simulink model "psbthermal"  (Simulink 6.0)
settings: Solver=ode23tb  StartTime=0.0  StopTime=0.5  MaxStep=50e-6  RelTol=1e-3
InitFcn:
  | powericon('psbinitsys',bdroot);
undefined symbols (not defined in the file or in its folder): D1, Delta
libraries: powerlib2 x31, powerlib_extras x1
settings Model: Creator=rchampag  LastModifiedBy=batserve  ExtModeTrigMode=oneshot  ExtModeArmWhenConnect=off  ExtModeAutoUpdateStatusClock=off
settings DataIOCC: LimitDataPoints=off  SaveOutput=off  SaveTime=off  TimeSaveName=t  SignalLoggingName=sigsOut
settings OptimizationCC: BlockReduction=off  BooleanDataType=off
settings DebuggingCC: CheckExecutionContextPreStartOutputMsg=on  CheckExecutionContextRuntimeOutputMsg=on  SolverPrmCheckMsg=none
settings HardwareCC: TargetUnknown=on

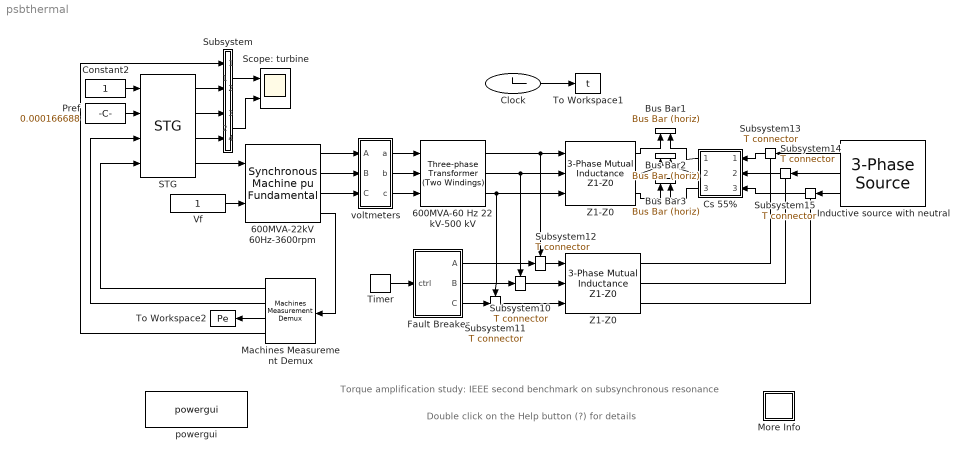
== system psbthermal ==
  note: Torque amplification study:
      | IEEE second benchmark on subsynchronous resonance
  note: Double click on the Help button (?) for details
  600MVA-22kV 60Hz-3600rpm : powerlib2/Machines/Synchronous Machine pu Fundamental  Tag=PoWeRsYsTeMbLoCk  rotorType=Round  x1="[ 600e6  22e3   60 ]"  x2="[  0.0045  0.14  1.51  1.45 ]"  x3="[  0.00096  0.1186 ]"  x4b="[ 0.016  0.132  0.00898  0.411  0.0116  0.0738 ]"  x4="[ 1.1685E-02  0.18167  1.9718E-02  038371 ]"  x5="[ 0.87882   0.176*8   1 ]"  x6="[0  0   0 0 0   0 0 0   0]"  x7=off  x8=[0.6404,0.7127,0.8441,0.9214,0.9956,1.082,1.19,1.316,1.457;0.7,0.7698,0.8872,0.9466,0.9969,1.046,1.1,1.151,1.201]  PSBOutputType=1110  iounits=0  LoadFlowParameters=[1 100000 0 0]
  600MVA-60 Hz 22 kV-500 kV : powerlib2/Elements/Three-phase Transformer (Two Windings)  Tag=PoWeRsYsTeMbLoCk  nominal="[ 600e6   60 ]"  type1=Delta (D1)  params1="[ 22e3  1e-6   0  ]"  type2=Yg  params2="[ 500e3  0.0012   0.12 ]"  ynsat=off  rmag=500  lm=500  sat="[ 0,0  ;  0.005,1.2  ;  1.0,1.4 ]"  hyst=off  matfile='hysteresis'  sif=off  phi0=[ 0.8 , -0.8 , 0.7 ]  initialslopes=[+1 +1 +1]  mesure=None  PSBOutputType=1111
  Bus Bar1 : powerlib2/Connectors/Bus Bar (horiz)  Tag=PoWeRsYsTeMbLoCk  Orientation=up  entrees=2  sorties=0  PSBOutputType=1111111111111111111111111111111111111111111111111111111111111111111111111
  Bus Bar2 : powerlib2/Connectors/Bus Bar (horiz)  Tag=PoWeRsYsTeMbLoCk  Orientation=up  entrees=2  sorties=0  PSBOutputType=1111111111111111111111111111111111111111111111111111111111111111111111111
  Bus Bar3 : powerlib2/Connectors/Bus Bar (horiz)  Tag=PoWeRsYsTeMbLoCk  Orientation=up  entrees=2  sorties=0  PSBOutputType=1111111111111111111111111111111111111111111111111111111111111111111111111
  Clock : Clock
      settings: Decimation=100
  Constant2 : Constant
  Cs 55% : Subsystem  Orientation=left
      mask Display: plot(0,0,100,100,[40,10],[50,50],[90,60],[50,50],[40,40],[20,80],[60,60],[20,80])
  Fault Breaker : Subsystem
  Inductive source with neutral : powerlib2/Electrical Sources/3-Phase Source  Tag=PoWeRsYsTeMbLoCk  Orientation=left  V=500e3  Phi=0  F=60  InternalConnection=Yg  RLoff=off  R=3.5  L=0.1989  Psc=0  Vbase=0  XRratio=0  PSBOutputType=111
  Machines Measurement Demux : powerlib2/Machines/Machines Measurement Demux  Orientation=left  machType=Synchronous  ssm1=on  ssm2=on  ssm3=on  ssm4=on  ssm5=on  ssm6=on  sm1=off  sm2=off  sm3=off  sm4=off  sm5=off  sm6=off  sm7=on  sm8=on  sm9=on  sm10=on  sm11=off  sm115=off  sm12=off  sm13=off  sm14=off  asm1=on  asm2=on  asm3=on  asm4=on  asm5=on  asm6=on  asm7=on  asm8=on  asm9=on  asm10=on  asm11=on  pmsm1=on  pmsm2=on  pmsm3=on  pmsm4=on  pmsm5=on  pmsm6=on  lastType=2
  More Info : Subsystem
      mask Display: disp('?')
  Pref : Constant  Value=0.000166688
  STG : powerlib2/Machines/STG  gentype=Tandem-compound (multi-mass)  reg1="[ 1  0.05    0 ]"  reg2="[ 0.001  0.15 ]"  reg3="[ -0.1  0.1  0.00016668  0.00016668*1.01 ]"  turb1="[ 0  10   3.3   0.5   ]"  turb2="[ 0.5   0.5   0  0 ]"  HA="[  1.5498   0.24894  0  0 ]"  KA="[  83.47  42.702  0  0 ]"  DA="[  0.3104  0.05  0  0 ]*8"  ini1=250.35/555  ini2=[0.000166688,-120.04]
  Scope: turbine : Scope  NumInputPorts=2
      settings: TimeRange=0.5  YMin=-0.9~-70  YMax=0.6~130
  Subsystem : Subsystem
  Subsystem10 : powerlib2/Connectors/T connector  Tag=PoWeRsYsTeMbLoCk  PSBOutputType=1
  Subsystem11 : powerlib2/Connectors/T connector  Tag=PoWeRsYsTeMbLoCk  PSBOutputType=1
  Subsystem12 : powerlib2/Connectors/T connector  Tag=PoWeRsYsTeMbLoCk  PSBOutputType=1
  Subsystem13 : powerlib2/Connectors/T connector  Tag=PoWeRsYsTeMbLoCk  Orientation=left  PSBOutputType=1
  Subsystem14 : powerlib2/Connectors/T connector  Tag=PoWeRsYsTeMbLoCk  Orientation=left  PSBOutputType=1
  Subsystem15 : powerlib2/Connectors/T connector  Tag=PoWeRsYsTeMbLoCk  Orientation=left  PSBOutputType=1
  Timer : powerlib_extras/Control  Blocks/Timer  t="[ 0.022289  0.022289+0.017 ]"  e=[ 1 0 ]
  To Workspace1 : ToWorkspace  VariableName=t  SaveFormat=Array
  To Workspace2 : ToWorkspace  VariableName=Pe  SaveFormat=Array
  Vf : Constant
  Z1-Z0 : powerlib2/Elements/3-Phase Mutual Inductance Z1-Z0  RL1="[ 18.5  0.5305 ]"  RL0="[ 55.0  1.5915 ]"
  "Z1-Z0 " : powerlib2/Elements/3-Phase Mutual Inductance Z1-Z0  RL1="[ 16.75  0.4901 ]"  RL0="[ 46.5  1.3926 ]"
  powergui : powerlib2/powergui  Frange=logspace(0,3,50)  Ylog=off  Xlog=off  save=off  variable=ZData  ZoomFFT=on  StartTime=0.0  cycles=2  DisplayStyle=off  fundamental=60  FreqAxis=off  MaxFrequency=1000  frequencyindice=1  frequencyindicesteady=1  RmsSteady=1  display=off  Ts=0  methode=off  frequency=60  echomessages=off
  voltmeters : Subsystem
  wires:
  Constant2/1 -> STG/1
  Machines Measurement Demux/1 -> STG/4
  Pref/1 -> STG/2
  Vf/1 -> 600MVA-22kV 60Hz-3600rpm/2
  600MVA-22kV 60Hz-3600rpm/4 -> Machines Measurement Demux/1
  STG/1 -> Subsystem/2(In2)
  Subsystem/2(Out2) -> Scope: turbine/2
  Machines Measurement Demux/2 -> STG/3
  Machines Measurement Demux/4 -> Subsystem/1(In1)
  Subsystem/1(Out1) -> Scope: turbine/1
  STG/2 -> Subsystem/3(In3)
  Machines Measurement Demux/3 -> To Workspace2/1
  Timer/1 -> Fault Breaker/1(ctrl)
  600MVA-22kV 60Hz-3600rpm/1 -> voltmeters/1(A)
  voltmeters/1(a) -> 600MVA-60 Hz 22 kV-500 kV/1
  600MVA-22kV 60Hz-3600rpm/2 -> voltmeters/2(B)
  voltmeters/2(b) -> 600MVA-60 Hz 22 kV-500 kV/2
  600MVA-22kV 60Hz-3600rpm/3 -> voltmeters/3(C)
  voltmeters/3(c) -> 600MVA-60 Hz 22 kV-500 kV/3
  Z1-Z0/1 -> Bus Bar1/1
  Z1-Z0/2 -> Bus Bar2/1
  Z1-Z0/3 -> Bus Bar3/1
  Inductive source with neutral/3 -> Subsystem15/1
  600MVA-60 Hz 22 kV-500 kV/2 -> Z1-Z0/2, Subsystem10/Enable
  600MVA-60 Hz 22 kV-500 kV/3 -> Z1-Z0/3, Subsystem11/Enable
  Subsystem12/1 -> "Z1-Z0 "/1
  Subsystem10/1 -> "Z1-Z0 "/2
  Subsystem11/1 -> "Z1-Z0 "/3
  600MVA-60 Hz 22 kV-500 kV/1 -> Subsystem12/Enable, Z1-Z0/1
  Fault Breaker/1(A) -> Subsystem12/1
  Fault Breaker/2(B) -> Subsystem10/1
  Fault Breaker/3(C) -> Subsystem11/1
  Cs 55%/1(Out1) -> Bus Bar1/2
  Cs 55%/2(Out2) -> Bus Bar2/2
  Cs 55%/3(Out3) -> Bus Bar3/2
  Inductive source with neutral/2 -> Subsystem14/1
  "Z1-Z0 "/3 -> Subsystem15/Enable
  "Z1-Z0 "/2 -> Subsystem14/Enable
  Subsystem14/1 -> Cs 55%/2(In2)
  Subsystem15/1 -> Cs 55%/3(In4)
  Subsystem13/1 -> Cs 55%/1(In1)
  Inductive source with neutral/1 -> Subsystem13/1
  Clock/1 -> To Workspace1/1
  STG/3 -> Subsystem/4(In4)
  STG/4 -> 600MVA-22kV 60Hz-3600rpm/1
  "Z1-Z0 "/1 -> Subsystem13/Enable

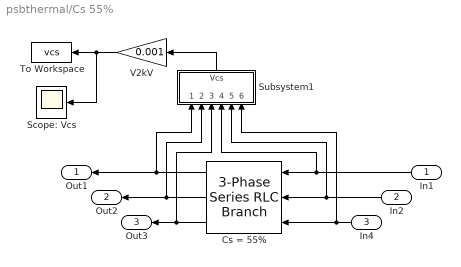
== system psbthermal/Cs 55% ==
  In1 : Inport  Orientation=left  Port=1  LatchInput=off
  In2 : Inport  Orientation=left  Port=2  LatchInput=off
  In4 : Inport  Orientation=left  Port=3  LatchInput=off
  Cs = 55% : powerlib2/Elements/3-Phase Series RLC Branch   Orientation=left  R=0  L=0  C=1/(0.55*0.5305*(120*pi)^2)
  Scope: Vcs : Scope
      settings: YMin=-500  YMax=500
  Subsystem1 : Subsystem  Orientation=up
  To Workspace : ToWorkspace  VariableName=vcs  SaveFormat=Array
  V2kV : Gain  Orientation=left  Gain=0.001  SaturateOnIntegerOverflow=on
  Out1 : Outport  Orientation=left
  Out2 : Outport  Orientation=left  Port=2
  Out3 : Outport  Orientation=left  Port=3
  wires:
  Cs = 55%/1 -> Subsystem1/1(A+), Out1/1
  Cs = 55%/2 -> Subsystem1/2(B+), Out2/1
  Cs = 55%/3 -> Subsystem1/3(C+), Out3/1
  In2/1 -> Cs = 55%/2, Subsystem1/5(B -)
  In4/1 -> Cs = 55%/3, Subsystem1/6(C -)
  Subsystem1/1(Vcs) -> V2kV/1
  In1/1 -> Cs = 55%/1, Subsystem1/4(A -)
  V2kV/1 -> To Workspace/1, Scope: Vcs/1

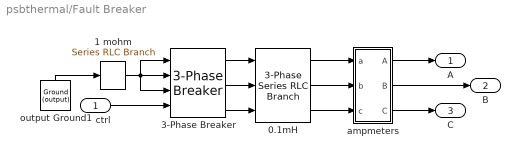
== system psbthermal/Fault Breaker ==
  ctrl : Inport  Port=1  LatchInput=off
  0.1mH : powerlib2/Elements/3-Phase Series RLC Branch   R=0  L=0.1e-3  C=inf
  1 mohm : powerlib2/Elements/Series RLC Branch  Tag=PoWeRsYsTeMbLoCk  a=0.001  b=0  c=inf  mesure=None  PSBOutputType=1
  3-Phase Breaker : powerlib2/Elements/3-Phase Breaker  init_states=open  sa=on  sb=on  sc=on  sw_times="[4/60  10/60]"  Ts=0  comext=on  Ron=0.001  Rp=1e6  Cp=inf  mesure=None
  ampmeters : Subsystem
  output Ground1 : powerlib2/Connectors/Ground (output)  Tag=PoWeRsYsTeMbLoCk  Orientation=up  PSBOutputType=1
  A : Outport
  B : Outport  Port=2
  C : Outport  Port=3
  wires:
  3-Phase Breaker/1 -> 0.1mH/1
  3-Phase Breaker/2 -> 0.1mH/2
  3-Phase Breaker/3 -> 0.1mH/3
  0.1mH/3 -> ampmeters/3(c)
  0.1mH/2 -> ampmeters/2(b)
  0.1mH/1 -> ampmeters/1(a)
  ctrl/1 -> 3-Phase Breaker/4
  ampmeters/1(A) -> A/1
  ampmeters/2(B) -> B/1
  ampmeters/3(C) -> C/1
  output Ground1/1 -> 1 mohm/1
  1 mohm/1 -> 3-Phase Breaker/3, 3-Phase Breaker/2, 3-Phase Breaker/1

== system psbthermal/More Info ==
  note: This system is an IEEE benchmark [1] used to study subsynchronous resonance and particularly torque amplification
      | after a fault on a series-compensated power system. It consists in a single generator (600 MVA/22kV/60 Hz/3600 rpm)
      | connected to an infinite bus via two transmission lines, one of which is series-compensated. The subsynchronous
      | mode introduced by the compensation capacitor after a fault has been applied and cleared excites the oscillatory
      | torsional modes of the multi-mass shaft and the torque amplification phenomenon can be observed.
  note: This demonstration illustrates subsynchronous resonance (SSR)
      | using the Steam Turbine and Governor on a series-compensated network
  note: Circuit Description
  note: Demonstration
  note: Reference
  note: [1] IEEE Subsynchronous resonance working group, "Second benchmark model for computer simulation of subsynchronous
      |      resonance", IEEE Transactions on power apparatus and systems, vol. PAS-104, no. 5, 1985, pp. 1057-1066.
  note: Louis-A. Dessaint and R. Champagne (Ecole de Technologie Superieure, Montreal)
  note: Open the Scope connected to the STG model. Run the simulation by selecting Start from the Simulation menu.
      | Observe the speed deviations on the top axis of the Scope and the torques transmitted between the shaft's
      | masses on the bottom axis. A peak torque of over 4 pu is observed between masses 1 and 2. The frequency
      | of the oscillations oberved in the torques and speed deviations is about 27 Hz. Excellent aggreement between
      | peak values observed here and those given in [1] is obtained.
  note: 1
  note: Open the synchronous machine (SM) block menu and observe that the machine intial conditions (last line)  are set to zero.
      | Start Simulation. As the SM initial conditions are not properly set you will observe that simulation does not start in steady state.
      | Stop the simulation.
  note: 2
  note: In order to start the simulation in steady-state you must initialize the synchronous machine for the desired load flow.
      | Open the  POWERGUI and select "Load Flow & Machine initialization" . The machine "Bus type" should be already initialized as "PV generator",
      | indicating that  the load flow will be performed with the machine controlling its active power and terminal voltage.
      | Specify the desired values by entering the following parameters:
  note: Load Flow: U AB (Vrms) = 22000 , P (wattts) =100e3
  note: Then press the "Update Load Flow" button.
      |
      | Once the load flow is solved the phasors of AB and BC machine voltages and currents flowing in phases A and B are updated.
      | The SM reactive power,  mechanical power and  field voltage are displayed : Q = 1.30 Mvar, Pmec = 100 kW (0.0001667 pu), field voltage Ef = 1.0036 pu;
      | If you open the SM block menu you will observe that the initial conditions have been updated.
  note: In order to start the simulation in steady state with the STG connected, this Simulink block must also be initialized according to the values
      | calculated by the load flow. This initialization is automatically performed when you execute the Load Flow, as long as you connect  at
      | the Pm and Vf inputs of the machine either Constant blocks or regulation blocks from the machine library (HTG, STG, or Excitation System).
      | Open the STG block menu and notice that the initial mechanical power and generator rotor angle have been automatically set to
      | Pm0=0.0001667 pu  (100.01 kW) and th0 = -120.04 degrees by the Load Flow. The Vf constant block connected at the Vf excitation input of the synchronous
      | machine has been automaticlly set to 1.00358 pu by the Load Flow. The Pref constant block connected at the Pref input of the STG block
      | has also been updated.
  note: 3
  note: 4

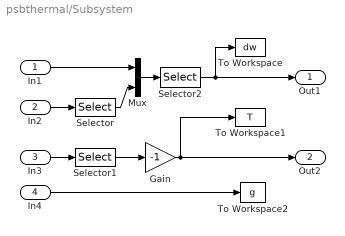
== system psbthermal/Subsystem ==
  In1 : Inport  Port=1  LatchInput=off
  In2 : Inport  Port=2  LatchInput=off
  In3 : Inport  Port=3  LatchInput=off
  In4 : Inport  Port=4  LatchInput=off
  Gain : Gain  Gain=-1  SaturateOnIntegerOverflow=on
  Mux : Mux  Inputs=2
  Selector : Selector  Elements=[3 4]  InputPortWidth=4
  Selector1 : Selector  Elements=[3 4]  InputPortWidth=4
  Selector2 : Selector  Elements=[2 3 1]  InputPortWidth=3
  To Workspace : ToWorkspace  VariableName=dw  SaveFormat=Array
  To Workspace1 : ToWorkspace  VariableName=T  SaveFormat=Array
  To Workspace2 : ToWorkspace  VariableName=g  SaveFormat=Array
  Out1 : Outport
  Out2 : Outport  Port=2
  wires:
  Selector/1 -> Mux/2
  Mux/1 -> Selector2/1
  In1/1 -> Mux/1
  In2/1 -> Selector/1
  In3/1 -> Selector1/1
  Selector2/1 -> Out1/1, To Workspace/1
  In4/1 -> To Workspace2/1
  Selector1/1 -> Gain/1
  Gain/1 -> To Workspace1/1, Out2/1

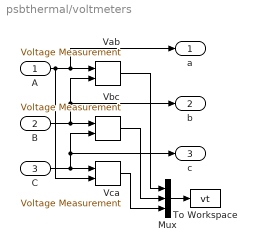
== system psbthermal/voltmeters ==
  A : Inport  Port=1  LatchInput=off
  B : Inport  Port=2  LatchInput=off
  C : Inport  Port=3  LatchInput=off
  Mux : Mux  Inputs=3
  To Workspace : ToWorkspace  VariableName=vt  SaveFormat=Array
  Vab : powerlib2/Measurements/Voltage Measurement  Tag=PoWeRsYsTeMmEaSuReMeNt  PhasorSimulation=off  OutputType=Magnitude  PSBOutputType=0  PSBequivalent=0
  Vbc : powerlib2/Measurements/Voltage Measurement  Tag=PoWeRsYsTeMmEaSuReMeNt  PhasorSimulation=off  OutputType=Magnitude  PSBOutputType=0  PSBequivalent=0
  Vca : powerlib2/Measurements/Voltage Measurement  Tag=PoWeRsYsTeMmEaSuReMeNt  PhasorSimulation=off  OutputType=Magnitude  PSBOutputType=0  PSBequivalent=1
  a : Outport
  b : Outport  Port=2
  c : Outport  Port=3
  wires:
  Vca/1 -> Mux/3
  Vbc/1 -> Mux/2
  Vab/1 -> Mux/1
  Mux/1 -> To Workspace/1
  B/1 -> Vbc/1, Vab/2, b/1
  C/1 -> Vca/1, Vbc/2, c/1
  A/1 -> Vab/1, a/1, Vca/2

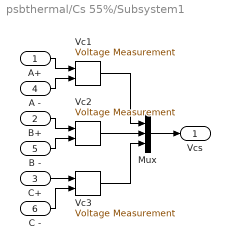
== system psbthermal/Cs 55%/Subsystem1 ==
  A+ : Inport  Port=1  LatchInput=off
  B+ : Inport  Port=2  LatchInput=off
  C+ : Inport  Port=3  LatchInput=off
  A - : Inport  Port=4  LatchInput=off
  B - : Inport  Port=5  LatchInput=off
  C - : Inport  Port=6  LatchInput=off
  Mux : Mux  Inputs=3
  Vc1 : powerlib2/Measurements/Voltage Measurement  Tag=PoWeRsYsTeMmEaSuReMeNt  PhasorSimulation=off  OutputType=Magnitude  PSBOutputType=0  PSBequivalent=0
  Vc2 : powerlib2/Measurements/Voltage Measurement  Tag=PoWeRsYsTeMmEaSuReMeNt  PhasorSimulation=off  OutputType=Magnitude  PSBOutputType=0  PSBequivalent=0
  Vc3 : powerlib2/Measurements/Voltage Measurement  Tag=PoWeRsYsTeMmEaSuReMeNt  PhasorSimulation=off  OutputType=Magnitude  PSBOutputType=0  PSBequivalent=0
  Vcs : Outport
  wires:
  C+/1 -> Vc3/1
  C -/1 -> Vc3/2
  Vc1/1 -> Mux/1
  Vc2/1 -> Mux/2
  Vc3/1 -> Mux/3
  Mux/1 -> Vcs/1
  B+/1 -> Vc2/1
  B -/1 -> Vc2/2
  A+/1 -> Vc1/1
  A -/1 -> Vc1/2

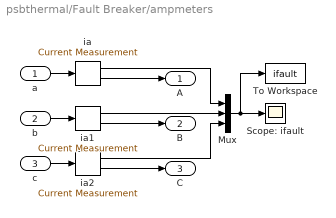
== system psbthermal/Fault Breaker/ampmeters ==
  a : Inport  Port=1  LatchInput=off
  b : Inport  Port=2  LatchInput=off
  c : Inport  Port=3  LatchInput=off
  Mux : Mux  Inputs=3
  Scope: ifault : Scope
      settings: YMin=-9000  YMax=9000
  To Workspace : ToWorkspace  VariableName=ifault  SaveFormat=Array
  ia : powerlib2/Measurements/Current Measurement  Tag=PoWeRsYsTeMmEaSuReMeNt  PhasorSimulation=off  OutputType=Magnitude  PSBOutputType=01  PSBequivalent=0
  ia1 : powerlib2/Measurements/Current Measurement  Tag=PoWeRsYsTeMmEaSuReMeNt  PhasorSimulation=off  OutputType=Magnitude  PSBOutputType=01  PSBequivalent=0
  ia2 : powerlib2/Measurements/Current Measurement  Tag=PoWeRsYsTeMmEaSuReMeNt  PhasorSimulation=off  OutputType=Magnitude  PSBOutputType=01  PSBequivalent=0
  A : Outport
  B : Outport  Port=2
  C : Outport  Port=3
  wires:
  a/1 -> ia/1
  b/1 -> ia1/1
  c/1 -> ia2/1
  ia/2 -> A/1
  ia1/2 -> B/1
  ia2/2 -> C/1
  ia/1 -> Mux/1
  ia1/1 -> Mux/2
  ia2/1 -> Mux/3
  Mux/1 -> Scope: ifault/1, To Workspace/1
